simulink model "four"  (R2019b)
settings: Solver=VariableStepAuto  StartTime=0.0  StopTime=10.0  RelTol=1e-3
settings Model: Creator=Pranshu  LastModifiedBy=Pranshu

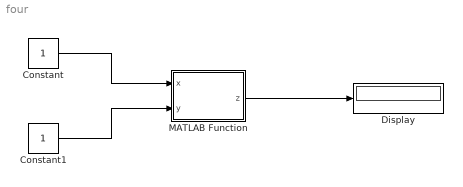
== system four ==
  Constant : Constant
  Constant1 : Constant
  Display : Display
  MATLAB Function : MATLAB Function  TreatAsAtomicUnit=on
  wires:
  Constant/1 -> MATLAB Function/1(x)
  Constant1/1 -> MATLAB Function/2(y)
  MATLAB Function/1(z) -> Display/1

== matlab function four/MATLAB Function ==
  data: x input; z output; y input
function z = fcn(x, y)

z = x+y;
